simulink model "ECUSIMLONK"  (R2024a)
settings: Solver=VariableStepAuto  StartTime=0.0  StopTime=10.0  RelTol=1e-3
settings Model: ExtModeTrigDuration=100  Creator=ABDERRAZEK  LastModifiedBy=ABDERRAZEK
settings DataIOCC: StateSaveName=tmp_raccel_xout
settings OptimizationCC: EfficientMapNaN2IntZero=off
settings DebuggingCC: ModelReferenceSymbolNameMessage=none
settings HardwareCC: TargetBitPerPointer=64  TargetBitPerSizeT=64  TargetBitPerPtrDiffT=64  TargetLongLongMode=on  TargetIntDivRoundTo=Zero  TargetEndianess=LittleEndian  TargetWordSize=64  TargetHWDeviceType=MATLAB Host  ProdEqTarget=off
settings SFSimCC: SimCustomCompilerFlags=-std=c++17  SimTargetLang=C++
settings RTWCC: SystemTargetFile=raccel.tlc  TemplateMakefile=raccel_default_tmf  RTWVerbose=off  RTWUseSimCustomCode=on  CustomBLASCallback=coder.internal.blas.MATLABBLASCallback  TargetLang=C++  DLTargetLibrary=mkl-dnn
settings CodeAppCC: GenerateComments=off  MaxIdLength=128  MangleLength=10  SimulinkBlockComments=off
settings RaccelTargetCC: TargetLangStandard=C++11 (ISO)  InstructionSetFMA=off  OptimizeReductions=off  LogToMDFFile=off  ENABLE_SLEXEC_SSBRIDGE=1  RTWCAPIParams=on  RTWCAPIRootIO=on

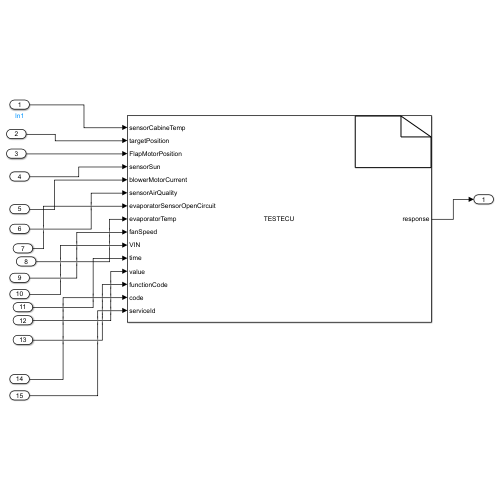
[thumbnail: Simulink's stored preview of the top-level diagram]
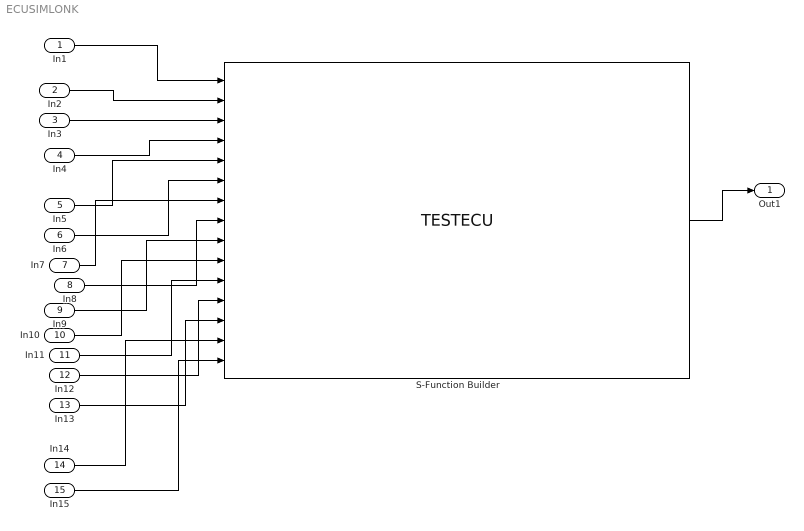
== system ECUSIMLONK ==
  In1 : Inport
  In2 : Inport  Port=2
  In3 : Inport  Port=3
  In4 : Inport  Port=4
  In5 : Inport  Port=5
  In6 : Inport  Port=6
  In7 : Inport  Port=7
  In8 : Inport  Port=8
  In9 : Inport  Port=9
  In10 : Inport  Port=10
  In11 : Inport  Port=11
  In12 : Inport  Port=12
  In13 : Inport  Port=13
  In14 : Inport  Port=14
  In15 : Inport  Port=15
  S-Function Builder : S-Function  FunctionName=TESTECU  SFunctionModules=TESTECU_wrapper.cpp  SFunctionDeploymentMode=off  EnableBusSupport=off  mask(S-Function Builder){}
      mask help: Simulink:masks:SFunctionBuilder_MD
      mask init:
      | val = [[.9  0.75 0.75 1 1 .9 .9 1]',[1 1 0.75 0.75 .9 .9 1 .9]'];try , sys = get_param(gcb,'SfunBuilderFcnName');if isempty(sys), sys = get_param(gcb,'FunctionName'); end,catch, sys = get_param(gcb,'FunctionName'); end
      settings: CopyFcn=set_param(gcbh,'LinkStatus','none')  OpenFcn=sfunctionwizard(gcbh)
      mask Display: plot(val(:,1),val(:,2)),disp(sys),port_label('input',1,'sensorCabineTemp'),port_label('input',2,'targetPosition'),port_label('input',3,'FlapMotorPosition'),port_label('input',4,'sensorSun'),port_label('input',5,'blowerMotorCurrent'),port_label('input',6,'sensorAirQuality'),port_label('input',7,'evaporatorSensorOpenCircuit'),port_label('input',8,'evaporatorTemp'),port_label('input',9,'fanSpeed'),port_label('input',10,'VIN'),port_label('input',11,'time'),port_label('input',12,'value'),port_label('input',13,'functionCode'),port_label('input',14,'code'),port_label('input',15,'serviceId'),port_label('output',1,'response')
  Out1 : Outport
  wires:
  In1/1 -> S-Function Builder/1
  In2/1 -> S-Function Builder/2
  In3/1 -> S-Function Builder/3
  In4/1 -> S-Function Builder/4
  In5/1 -> S-Function Builder/5
  In6/1 -> S-Function Builder/6
  In7/1 -> S-Function Builder/7
  In8/1 -> S-Function Builder/8
  In9/1 -> S-Function Builder/9
  In10/1 -> S-Function Builder/10
  In11/1 -> S-Function Builder/11
  In12/1 -> S-Function Builder/12
  In13/1 -> S-Function Builder/13
  In14/1 -> S-Function Builder/14
  In15/1 -> S-Function Builder/15
  S-Function Builder/1 -> Out1/1
